simulink model "observernonlindesign"  (R2019b)
settings: Solver=VariableStepAuto  StartTime=0.0  StopTime=10.0  RelTol=1e-3
values from neighbouring files (symbols this model uses):
  A = [-1/9 1/9;1/9 -0.3889]    [lqrfeedback_params.m]    (also in observerbasednonlin_params.m = 0.01; observerdesign_params.m; statefeedback_params.m; statefeedbacknonlin_params.m = 0.01)
  A11 = A(1,1)    [lqrfeedback_params.m]    (also in observerbasednonlin_params.m = Ao(1,1); observerdesign_params.m; statefeedback_params.m)
  A12 = A(1,2)    [lqrfeedback_params.m]    (also in observerbasednonlin_params.m = Ao(1,2); observerdesign_params.m; statefeedback_params.m)
  A21 = A(2,1)    [lqrfeedback_params.m]    (also in observerbasednonlin_params.m = Ao(2,1); observerdesign_params.m; statefeedback_params.m)
  A22 = A(2,2)    [lqrfeedback_params.m]    (also in observerbasednonlin_params.m = Ao(2,2); observerdesign_params.m; statefeedback_params.m)
  B1 = B(1)    [lqrfeedback_params.m]    (also in observerbasednonlin_params.m; observerdesign_params.m; statefeedback_params.m)
  g = 9.81    [observerbasednonlin_params.m]    (also in statefeedbacknonlin_params.m)
  h1_init = 1    [observerbasednonlin_params.m]    (also in observerdesign_params.m = 0)
  h1eq = 0    [lqrfeedback_params.m]    (also in observerbasednonlin_params.m; observerdesign_params.m; statefeedback_params.m; statefeedbacknonlin_params.m)
  h2_init = 1    [observerbasednonlin_params.m]    (also in observerdesign_params.m)
  h2eq = 0    [lqrfeedback_params.m]    (also in observerbasednonlin_params.m; observerdesign_params.m; statefeedback_params.m; statefeedbacknonlin_params.m)
  k1 = k(1)    [lqrfeedback_params.m]    (also in observerbasednonlin_params.m = 1.095; observerdesign_params.m = 0.0151; statefeedback_params.m = 1.09; statefeedbacknonlin_params.m = 1.09)
  k2 = k(2)    [lqrfeedback_params.m]    (also in observerbasednonlin_params.m = 87.12; observerdesign_params.m = 0.3997; statefeedback_params.m = 86.1515; statefeedbacknonlin_params.m = 86.1515)
  Ke1 = 43.22    [observerbasednonlin_params.m]    (also in observerdesign_params.m = 9091)
  Ke2 = 1.5    [observerbasednonlin_params.m]    (also in observerdesign_params.m = 109.51)
  qeq = 0    [lqrfeedback_params.m]    (also in observerbasednonlin_params.m; observerdesign_params.m; statefeedback_params.m)
  ro = 1    [observerbasednonlin_params.m]    (also in statefeedbacknonlin_params.m)
  ro1 = 1.262*10e-4    (= 0.001262)    [observerbasednonlin_params.m]    (also in statefeedbacknonlin_params.m = 178.57)
  ro2 = 1.262*10e-4    (= 0.001262)    [observerbasednonlin_params.m]    (also in statefeedbacknonlin_params.m = 178.57)
settings Model: Creator=SAI JOSHITHA  LastModifiedBy=SAI JOSHITHA

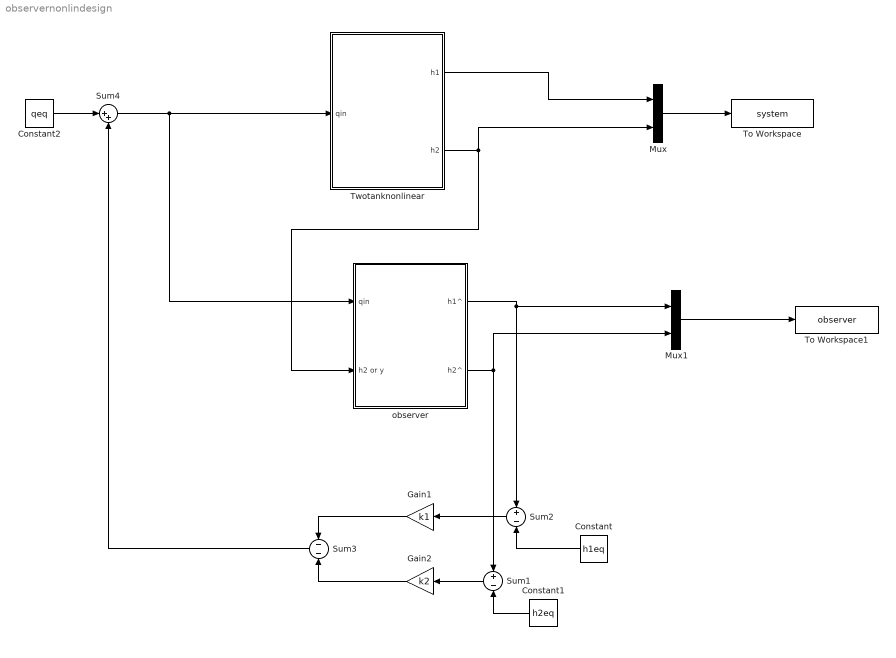
== system observernonlindesign ==
  Constant : Constant  Value=h1eq
  Constant1 : Constant  Value=h2eq
  Constant2 : Constant  Value=qeq
  Gain1 : Gain  Gain=k1
  Gain2 : Gain  Gain=k2
  Mux : Mux  Inputs=2
  Mux1 : Mux  Inputs=2
  Sum1 : Sum  Inputs=+-
  Sum2 : Sum  Inputs=+-
  Sum3 : Sum  Inputs=--
  Sum4 : Sum  Inputs=|++
  To Workspace : ToWorkspace  VariableName=system  SaveFormat=Timeseries  SampleTime=-1
  To Workspace1 : ToWorkspace  VariableName=observer  SaveFormat=Timeseries  SampleTime=-1
  Twotanknonlinear : Subsystem
  observer : Subsystem
  wires:
  Sum1/1 -> Gain2/1
  Mux1/1 -> To Workspace1/1
  Gain1/1 -> Sum3/1
  Twotanknonlinear/1(h1) -> Mux/1
  Mux/1 -> To Workspace/1
  Constant/1 -> Sum2/2
  observer/1(h1^) -> Sum2/1, Mux1/1
  Sum4/1 -> Twotanknonlinear/1(qin), observer/1(qin)
  Gain2/1 -> Sum3/2
  Twotanknonlinear/2(h2) -> Mux/2, observer/2(h2 or y)
  Constant1/1 -> Sum1/2
  observer/2(h2^) -> Sum1/1, Mux1/2
  Sum2/1 -> Gain1/1
  Constant2/1 -> Sum4/1
  Sum3/1 -> Sum4/2

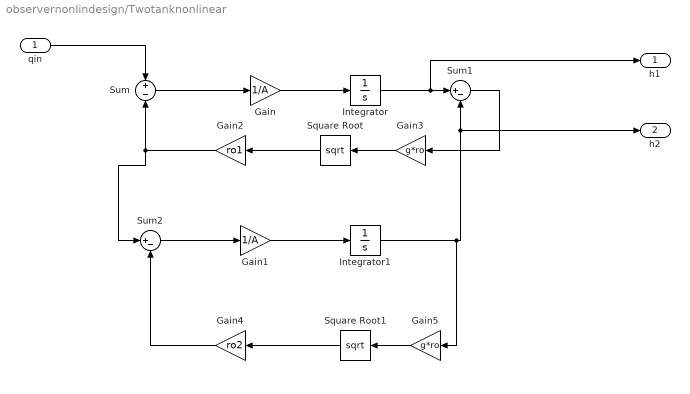
== system observernonlindesign/Twotanknonlinear ==
  qin : Inport
  Gain : Gain  Gain=1/A
  Gain1 : Gain  Gain=1/A
  Gain2 : Gain  Gain=ro1
  Gain3 : Gain  Gain=g*ro
  Gain4 : Gain  Gain=ro2
  Gain5 : Gain  Gain=g*ro
  Integrator : Integrator  InitialCondition=h1_init
  Integrator1 : Integrator  InitialCondition=h2_init
  Square Root : Sqrt  SaturateOnIntegerOverflow=on
  Square Root1 : Sqrt  SaturateOnIntegerOverflow=on
  Sum : Sum  Inputs=+-
  Sum1 : Sum  Inputs=|+-
  Sum2 : Sum  Inputs=|+-
  h1 : Outport
  h2 : Outport  Port=2
  wires:
  Gain3/1 -> Square Root/1
  Integrator/1 -> h1/1, Sum1/1
  Gain2/1 -> Sum2/1, Sum/2
  Sum2/1 -> Gain1/1
  Gain1/1 -> Integrator1/1
  Gain/1 -> Integrator/1
  Square Root/1 -> Gain2/1
  Sum/1 -> Gain/1
  Integrator1/1 -> Gain5/1, h2/1, Sum1/2
  Sum1/1 -> Gain3/1
  Square Root1/1 -> Gain4/1
  Gain5/1 -> Square Root1/1
  Gain4/1 -> Sum2/2
  qin/1 -> Sum/1

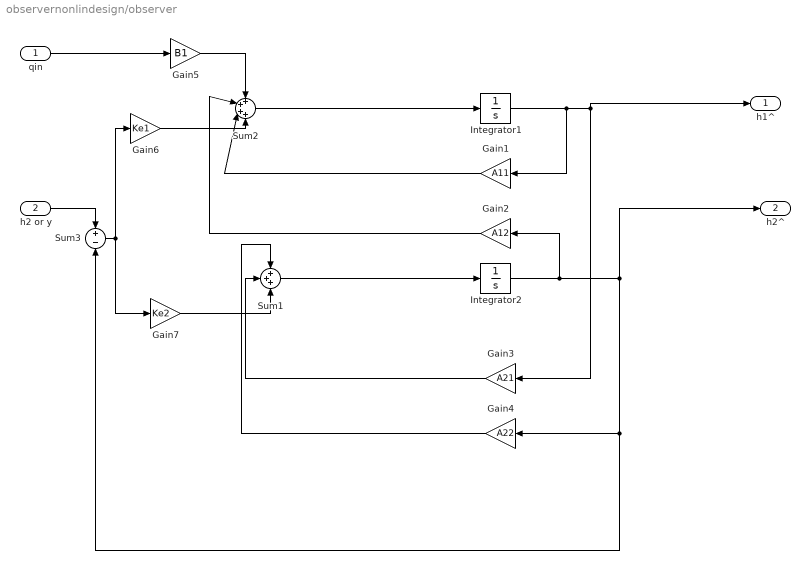
== system observernonlindesign/observer ==
  qin : Inport
  h2 or y : Inport  Port=2
  Gain1 : Gain  Gain=A11
  Gain2 : Gain  Gain=A12
  Gain3 : Gain  Gain=A21
  Gain4 : Gain  Gain=A22
  Gain5 : Gain  Gain=B1
  Gain6 : Gain  Gain=Ke1
  Gain7 : Gain  Gain=Ke2
  Integrator1 : Integrator  InitialCondition=h1_init
  Integrator2 : Integrator  InitialCondition=h2_init
  Sum1 : Sum  Inputs=+++
  Sum2 : Sum  Inputs=++++
  Sum3 : Sum  Inputs=+-
  h1^ : Outport
  h2^ : Outport  Port=2
  wires:
  Integrator2/1 -> Gain2/1, Sum3/2, Gain4/1, h2^/1
  Integrator1/1 -> Gain1/1, Gain3/1, h1^/1
  Gain3/1 -> Sum1/2
  Sum2/1 -> Integrator1/1
  Gain4/1 -> Sum1/1
  Gain2/1 -> Sum2/2
  Gain5/1 -> Sum2/1
  Sum1/1 -> Integrator2/1
  Gain1/1 -> Sum2/3
  qin/1 -> Gain5/1
  h2 or y/1 -> Sum3/1
  Sum3/1 -> Gain7/1, Gain6/1
  Gain6/1 -> Sum2/4
  Gain7/1 -> Sum1/3
